simulink model "ErrorHandling_v2"  (R2020a)
settings: Solver=VariableStepAuto  StartTime=0.0  StopTime=10.0  RelTol=1e-3  EnableMultiTasking=on
settings Model: Creator=Flanker  LastModifiedBy=Flanker
settings DataIOCC: LimitDataPoints=on  ReturnWorkspaceOutputs=off
settings OptimizationCC: LifeSpan=inf
settings DebuggingCC: AllowSymbolicDim=off  SFUnexpectedBacktrackingDiag=warning  SFNoUnconditionalDefaultTransitionDiag=warning  SFExecutionAtInitializationDiag=none  ArithmeticOperatorsInVariantConditions=warning
settings ModelReferenceCC: PropagateSignalLabelsOutOfModel=off
settings SFSimCC: SimUseLocalCustomCode=off  CustomCodeUndefinedFunction=UseInterfaceOnly
settings RTWCC: RTWUseLocalCustomCode=off
settings CodeAppCC: StateflowObjectComments=on
settings GRTTargetCC: TargetLangStandard=C89/C90 (ANSI)
settings ConfigComp: CovMetricSettings=dw  CovHtmlReporting=on  CovSaveCumulativeToWorkspaceVar=on  CovSaveSingleToWorkspaceVar=on  CovExternalEMLEnable=off

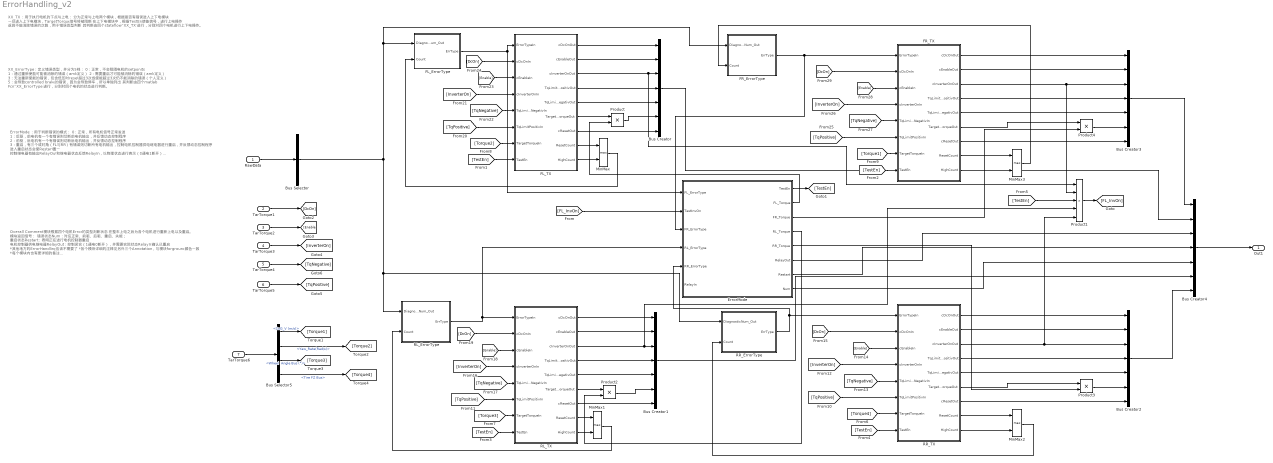
== system ErrorHandling_v2 ==
  note: XX_ErrorType ：定义错误类型，并分为5档：
      | 0：正常，不会阻隔电机的setponits
      | 1：通过重新使能可能被消除的错误（amk定义）
      | 2：需要重启才可能被消除的错误（amk定义）
      | 3：无法重新使能的错误，包含低压时reset超过3次或使能超过3次仍不能消除的错误（个人定义）
      | 5：会导致controlled brake的错误，因为会导致停车，所以单独列出
      |
      | 其判断由四个matlab Fcn“XX_ErrorType”进行，分别对四个电机的状态进行判断。
  note: XX_TX ：用于执行电机的下点与上电：
      | 分为正常与上电两个模块，根据是否有错误进入上下电模块
      | 一旦进入上下电模块，TargetTorque信号将被阻断
      | 在上下电模块中，根据TestEn使能信号，进行上电操作
      | 返回不能消除错误的次数，用于错误类型判断
      |
      | 其判断由四个stateflow“XX_TX”进行，分别对四个电机进行上下电操作。
  note: ErrorMode ：用于判断错误的模式：
      | 0：正常，所有电机信号正常发送
      | 1：后驱，前电机有一个有错误则切断前电机输出，并反馈动态控制程序
      | 2：前驱，后电机有一个有错误则切断后电机输出，并反馈动态控制程序
      | 3：重启，有三个或对角（FL与RR）有错误则切断所有电机输出，控制电机控制器供电继电器进行重启，并反馈动态控制程序
      | 进入重启状态会使Restart置一
      | 控制继电器有输出RelayOut和继电器状态反馈RelayIn，以物理状态进行表示（0通电1断开）
      | 电机控制器重新上电后，TestEn置一，控制TX模块进行电机上电
      | 4：失能，重启次数超过3次仍不能解除错误状态，则停止重启的状态，并反馈动态控制程序
      |
      | 会根据所在模式，切断TargetTorque信号
      |
      | 其判断由stateflow“ErrorMode”进行，分别对四个电机进行上下电操作。
  note: Overall Comment
      |
      | 模块根据四个电机Error的类型判断状态
      | 在整车上电之后为各个电机进行重新上电以及重启。
      |
      | 模块返回信号：
      |
      | 错误状态Num：对应正常、前驱、后驱、重启、失能；
      | 重启状态Restart：表明正在进行电机控制器重启
      | 电机控制器供电继电器RelayOut：控制闭合（1通电0断开），并需要实际状态RelayIn确认已重启
      |
      | *其他地方的ErrorHandling应该不需要了
      | *各个模块详细的注释见另外三个Annotation，与模块forground颜色一致
      | *每个模块内也有更详细的备注
      | *很多错误没有出现过，也没看懂到底怎么解决，所以归类方式以结果为主，并没有更深入的进行handling
      | *其实很多错误根本无法在行驶中被消除，但是垂死挣扎，此程序主要意义还是切换前驱后驱
      |
      | 2020/2/6 V2.0
  RawData : Inport
  TarTorque1 : Inport  Port=2
  TarTorque2 : Inport  Port=3
  TarTorque3 : Inport  Port=4
  TarTorque4 : Inport  Port=5
  TarTorque5 : Inport  Port=6
  TarTorque6 : Inport  Port=7
  Bus Creator{,1..4} (5 alike) : BusCreator  Inputs=7
  Bus Selector : BusSelector  OutputSignals=signal1,signal2  OutputAsBus=on
  Bus Selector5 : BusSelector  OutputSignals="processed data.CoG_V (m/s),processed data.Yaw_Rate(Rad/s),processed data.Wheel  Angle Bus (°),processed data.Tire FZ Bus"
  ErrorMode : Stateflow chart  TreatAsAtomicUnit=on
  FL_ErrorType : MATLAB Function  TreatAsAtomicUnit=on
  "FL_TX " : Stateflow chart  TreatAsAtomicUnit=on
  FR_ErrorType : MATLAB Function  TreatAsAtomicUnit=on
  FR_TX : Stateflow chart  TreatAsAtomicUnit=on
  MinMax{,1..3} (4 alike) : MinMax  Function=max  Inputs=2
  Product{,2..4} (4 alike) : Product
  Product1 : Product  Inputs=5
  RL_ErrorType : MATLAB Function  TreatAsAtomicUnit=on
  RL_TX : Stateflow chart  TreatAsAtomicUnit=on
  RR_ErrorType : MATLAB Function  TreatAsAtomicUnit=on
  RR_TX : Stateflow chart  TreatAsAtomicUnit=on
  Out1 : Outport
  wires:
  FL_ErrorType/1(ErrType) -> ErrorMode/1(FL_ErrorType), "FL_TX "/1(ErrorTypeIn)
  "FL_TX "/8(ResetCount) -> MinMax/1
  "FL_TX "/9(HighCount) -> MinMax/2
  MinMax/1 -> FL_ErrorType/2(Count)
  "FL_TX "/3(cInverterOnOut) -> Product1/1, Bus Creator/3
  "FL_TX "/1(cDcOnOut) -> Bus Creator/1
  "FL_TX "/2(cEnableOut) -> Bus Creator/2
  "FL_TX "/4(TqLimitPositivOut) -> Bus Creator/4
  "FL_TX "/5(TqLimitNegativOut) -> Bus Creator/5
  "FL_TX "/6(TargetTorqueOut) -> Product/1
  "FL_TX "/7(cResetOut) -> Bus Creator/7
  Product/1 -> Bus Creator/6
  [FL_InvOn] -> ErrorMode/2(TestInvOn)
  RawData/1 -> Bus Selector/1
  Product1/1 -> [FL_InvOn]
  RL_TX/3(cInverterOnOut) -> Product1/4, Bus Creator1/3
  RL_TX/1(cDcOnOut) -> Bus Creator1/1
  RL_TX/2(cEnableOut) -> Bus Creator1/2
  RL_TX/4(TqLimitPositivOut) -> Bus Creator1/4
  RL_TX/5(TqLimitNegativOut) -> Bus Creator1/5
  RL_TX/6(TargetTorqueOut) -> Product2/1
  RL_TX/7(cResetOut) -> Bus Creator1/7
  Product2/1 -> Bus Creator1/6
  RR_TX/3(cInverterOnOut) -> Bus Creator2/3, Product1/5
  RR_TX/1(cDcOnOut) -> Bus Creator2/1
  RR_TX/2(cEnableOut) -> Bus Creator2/2
  RR_TX/4(TqLimitPositivOut) -> Bus Creator2/4
  RR_TX/5(TqLimitNegativOut) -> Bus Creator2/5
  RR_TX/6(TargetTorqueOut) -> Product3/1
  RR_TX/7(cResetOut) -> Bus Creator2/7
  Product3/1 -> Bus Creator2/6
  FR_TX/3(cInverterOnOut) -> Bus Creator3/3, Product1/2
  FR_TX/1(cDcOnOut) -> Bus Creator3/1
  FR_TX/2(cEnableOut) -> Bus Creator3/2
  FR_TX/4(TqLimitPositivOut) -> Bus Creator3/4
  FR_TX/5(TqLimitNegativOut) -> Bus Creator3/5
  FR_TX/6(TargetTorqueOut) -> Product4/1
  FR_TX/7(cResetOut) -> Bus Creator3/7
  Product4/1 -> Bus Creator3/6
  FR_TX/8(ResetCount) -> MinMax3/1
  FR_TX/9(HighCount) -> MinMax3/2
  FR_ErrorType/1(ErrType) -> ErrorMode/3(FR_ErrorType), FR_TX/1(ErrorTypeIn)
  RL_TX/8(ResetCount) -> MinMax1/1
  RL_TX/9(HighCount) -> MinMax1/2
  RR_TX/8(ResetCount) -> MinMax2/1
  RR_TX/9(HighCount) -> MinMax2/2
  RR_ErrorType/1(ErrType) -> ErrorMode/5(RR_ErrorType), RR_TX/1(ErrorTypeIn)
  RL_ErrorType/1(ErrType) -> ErrorMode/4(RL_ErrorType), RL_TX/1(ErrorTypeIn)
  MinMax1/1 -> RL_ErrorType/2(Count)
  MinMax3/1 -> FR_ErrorType/2(Count)
  Bus Creator3/1 -> Bus Creator4/1
  Bus Creator/1 -> Bus Creator4/2
  Bus Creator1/1 -> Bus Creator4/6
  Bus Creator2/1 -> Bus Creator4/7
  Bus Creator4/1 -> Out1/1
  ErrorMode/1(TestEn) -> [TestEn]
  [TestEn] -> "FL_TX "/8(TestEn)
  [TestEn] -> FR_TX/8(TestEn)
  [TestEn] -> RL_TX/8(TestEn)
  [TestEn] -> Product1/3
  ErrorMode/2(FL_Torque) -> Product/2
  ErrorMode/3(FR_Torque) -> Product4/2
  ErrorMode/4(RL_Torque) -> Product2/2
  ErrorMode/5(RR_Torque) -> Product3/2
  ErrorMode/6(RelayOut) -> Bus Creator4/3
  ErrorMode/7(Restart) -> Bus Creator4/4
  Bus Selector/1 -> RL_ErrorType/1(DiagnosticNum_Out), RR_ErrorType/1(DiagnosticNum_Out), FR_ErrorType/1(DiagnosticNum_Out), FL_ErrorType/1(DiagnosticNum_Out)
  MinMax2/1 -> RR_ErrorType/2(Count)
  ErrorMode/8(Num) -> Bus Creator4/5
  TarTorque4/1 -> [TqNegative]
  TarTorque1/1 -> [DcOn]
  TarTorque2/1 -> [Enable]
  TarTorque3/1 -> [InverterOn]
  [TestEn] -> RR_TX/8(TestEn)
  TarTorque6/1 -> Bus Selector5/1
  Bus Selector5/2 -> [Torque2]  "<Yaw_Rate(Rad/s)>"
  Bus Selector5/1 -> [Torque1]  "<CoG_V (m/s)>"
  Bus Selector5/3 -> [Torque3]  "<Wheel  Angle Bus (°)>"
  Bus Selector5/4 -> [Torque4]  "<Tire FZ Bus>"
  [Torque4] -> RR_TX/7(TargetTorqueIn)
  [Torque3] -> RL_TX/7(TargetTorqueIn)
  [Torque2] -> "FL_TX "/7(TargetTorqueIn)
  [Torque1] -> FR_TX/7(TargetTorqueIn)
  TarTorque5/1 -> [TqPositive]
  [TqPositive] -> RR_TX/6(TqLimitPositivIn)
  [TqPositive] -> RL_TX/6(TqLimitPositivIn)
  [TqNegative] -> RR_TX/5(TqLimitNegativIn)
  [InverterOn] -> RR_TX/4(cInverterOnIn)
  [Enable] -> RR_TX/3(cEnableIn)
  [DcOn] -> RR_TX/2(cDcOnIn)
  [Enable] -> RL_TX/3(cEnableIn)
  [DcOn] -> RL_TX/2(cDcOnIn)
  [InverterOn] -> RL_TX/4(cInverterOnIn)
  [TqNegative] -> RL_TX/5(TqLimitNegativIn)
  [InverterOn] -> "FL_TX "/4(cInverterOnIn)
  [TqPositive] -> "FL_TX "/6(TqLimitPositivIn)
  [DcOn] -> "FL_TX "/2(cDcOnIn)
  [Enable] -> "FL_TX "/3(cEnableIn)
  [TqNegative] -> "FL_TX "/5(TqLimitNegativIn)
  [TqPositive] -> FR_TX/6(TqLimitPositivIn)
  [InverterOn] -> FR_TX/4(cInverterOnIn)
  [DcOn] -> FR_TX/2(cDcOnIn)
  [Enable] -> FR_TX/3(cEnableIn)
  [TqNegative] -> FR_TX/5(TqLimitNegativIn)

== stateflow chart ErrorHandling_v2/RL_TX ==
  state E1
    state S1
      en:
      TargetTorqueOut=0;
      TqLimitNegativOut=0;
      TqLimitPositivOut=0;
      n=0;
      du:
      n=n+1;
    state S8
      en:
      cInverterOn=1;
      n=0;
      du:
      n=n+1;
    state S2
      en:
      cInverterOnOut=0;
      n=0;
      du:
      n=n+1;
    state S7
      en:
      cEnableOut=1;
      n=0;
      du:
      n=n+1;
    state S3
      en:
      cEnableOut=0;
      n=0;
      du:
      n=n+1;
    state S6
      en:
      cDcOnOut=1;
      n=0;
      du:
      n=n+1;
    state S4
      en:
      cDcOnOut=0;
      n=0;
      du:
      n=n+1;
    state S5
      en:
      cReset=1;
      n=0;
      du:
      n=n+1;
      ex:
      cReset=0;
    (junction 68) -> S2 : HighCoun[ErrorTypeIn~=0]{HighCount = HighCount + 1;}
    S8 -> (junction 68) : [n>10]
    (default) -> S1
    S1 -> S2 : [n>5]
    S7 -> S8 : [n>5]
    S2 -> S3 : [n>5]
    S6 -> S7 : [n>5]
    (junction 85) -> S6 [order 2] : [TestEn==1]...
        | {HighCount=0;ResetCount=0;}
    S3 -> S4 : [n>5]
    (junction 43) -> S6 [order 1] : [ErrorTypeIn~=1]{ResetCount=0;}
    (junction 43) -> S5 [order 2] : ResetCoun[ErrorTypeIn==1&ResetCount<4]{ResetCount = ResetCount + 1;}
    (junction 43) -> (junction 85) [order 3] : [ResetCount==4]
    S5 -> (junction 43) : [n>10]
    S4 -> (junction 85) : [n>5]
  state E0
    en:
    ErrorState=ErrorTypeIn;
    ResetCount=0;
    HighCount=0;
    du:
    cDcOnOut=cDcOnIn;
    cEnableOut=cEnableIn;
    cInverterOnOut=cInverterOnIn;
    TqLimitPositivOut=TqLimitPositivIn;
    TqLimitNegativOut=TqLimitNegativIn;
    TargetTorqueOut=TargetTorqueIn;
    ex:
    ErrorState=ErrorTypeIn;
  note: TX ：用于执行电机的下电与上电：
      | 分为正常“E0”与上下电“E1”两个模块，根据是否有错误“ErrorTypeIn”进入上下电模块。
      | 一旦进入上下电模块，TqLimit以及TargetTorque信号将被阻断，并逐步下电。
      | 因为只有ErrorType=1时，下电再上电可能消除错误，其他错误类型（>1）将被限制在juncture处。
      | 当“ErrorMode”模块进行重启后，“TestEn”使上下电模块进行上电操作
      | “ResetCount”是低压错误重置失败次数，"HighCount"是使能后错误出现次数，两者将取最大值返回“XX_ErrorType”用于判断错误类型
      |
      | 注意：使用n计数可能导致命令送出时延过短（未成功送出），调试时需注意
  note: 
  (default) -> E0
  E0 -> E1 : [ErrorTypeIn~=0]
  E1 -> E0 : [ErrorTypeIn==0]
  (junction 85) -> S5 [order 1] : [ErrorTypeIn<2||HighCount<4]
  data: cDcOnOut output; ErrorTypeIn input; cDcOnIn input [0..1]; cEnableIn input [0..1]; cInverterOnIn input [0..1]; n local =0; cEnableOut output; cInverterOnOut output; TqLimitPositivOut output; TqLimitNegativOut output; TargetTorqueOut output; TqLimitNegativIn input; TqLimitPositivIn input; TargetTorqueIn input; cResetOut output; ErrorState local =0; ResetCount output =0; HighCount output =0; TestEn input

== matlab function ErrorHandling_v2/RL_ErrorType ==
  data: DiagnosticNum_Out input; ErrType output; Count input
function ErrType = ErrorType(DiagnosticNum_Out,Count)
    if DiagnosticNum_Out==0&&Count<4
        ErrType=0;%没有错误
    elseif (DiagnosticNum_Out==3587 || DiagnosticNum_Out==3585 ...
            ||MCFL_Diagnost==2310)&&Count<4
        ErrType=2;%错误需要软件重启
    elseif (DiagnosticNum_Out==1049 || DiagnosticNum_Out==1066 ...
            ||DiagnosticNum_Out==1101|| DiagnosticNum_Out==2360 ...
            ||DiagnosticNum_Out==2361|| DiagnosticNum_Out==2363 ...
            ||DiagnosticNum_Out==2364|| DiagnosticNum_Out==2365 ...
            ||DiagnosticNum_Out==2399)&&Count<4
        ErrType=4;%导致Controlled Brake的错误，停车进行硬件重启
    elseif DiagnosticNum_Out~=0&&Count>3
        ErrType=3;%无法重新使能的错误（由1、2产生）
    else
        ErrType = 1;%错误需要重新使能
    end
end
% 定义错误类型，并分为5档：
% 0：正常，不会阻隔电机的setponits
% 1：通过重新使能可能被消除的错误（amk定义），因为没被列举的错误极多，
% 很多没见过也不知如何处理，便用else归类
% 2：需要重启才可能被消除的错误（amk定义）
% 3：无法重新使能的错误，包含低压时reset超过3次或使能超过3次仍不能消除的错误（个人定义）
% 5：会导致controlled brake的错误，因为会导致停车，所以单独列出
% 
% 很多错误没有出现过，也没看懂到底怎么解决，所以归类方式以结果为主，并没有更深入的进行handling
% 其实很多错误根本无法在行驶中被消除，但是垂死挣扎，此程序主要意义还是切换前驱后驱

== stateflow chart ErrorHandling_v2/RR_TX ==
  state E1
    state S1
      en:
      TargetTorqueOut=0;
      TqLimitNegativOut=0;
      TqLimitPositivOut=0;
      n=0;
      du:
      n=n+1;
    state S8
      en:
      cInverterOn=1;
      n=0;
      du:
      n=n+1;
    state S2
      en:
      cInverterOnOut=0;
      n=0;
      du:
      n=n+1;
    state S7
      en:
      cEnableOut=1;
      n=0;
      du:
      n=n+1;
    state S3
      en:
      cEnableOut=0;
      n=0;
      du:
      n=n+1;
    state S6
      en:
      cDcOnOut=1;
      n=0;
      du:
      n=n+1;
    state S4
      en:
      cDcOnOut=0;
      n=0;
      du:
      n=n+1;
    state S5
      en:
      cReset=1;
      n=0;
      du:
      n=n+1;
      ex:
      cReset=0;
    (junction 68) -> S2 : HighCoun[ErrorTypeIn~=0]{HighCount = HighCount + 1;}
    S8 -> (junction 68) : [n>10]
    (default) -> S1
    S1 -> S2 : [n>5]
    S7 -> S8 : [n>5]
    S2 -> S3 : [n>5]
    S6 -> S7 : [n>5]
    (junction 85) -> S6 [order 2] : [TestEn==1]...
        | {HighCount=0;ResetCount=0;}
    S3 -> S4 : [n>5]
    (junction 43) -> S6 [order 1] : [ErrorTypeIn~=1]{ResetCount=0;}
    (junction 43) -> S5 [order 2] : ResetCoun[ErrorTypeIn==1&ResetCount<4]{ResetCount = ResetCount + 1;}
    (junction 43) -> (junction 85) [order 3] : [ResetCount==4]
    S5 -> (junction 43) : [n>10]
    S4 -> (junction 85) : [n>5]
  state E0
    en:
    ErrorState=ErrorTypeIn;
    ResetCount=0;
    HighCount=0;
    du:
    cDcOnOut=cDcOnIn;
    cEnableOut=cEnableIn;
    cInverterOnOut=cInverterOnIn;
    TqLimitPositivOut=TqLimitPositivIn;
    TqLimitNegativOut=TqLimitNegativIn;
    TargetTorqueOut=TargetTorqueIn;
    ex:
    ErrorState=ErrorTypeIn;
  note: TX ：用于执行电机的下电与上电：
      | 分为正常“E0”与上下电“E1”两个模块，根据是否有错误“ErrorTypeIn”进入上下电模块。
      | 一旦进入上下电模块，TqLimit以及TargetTorque信号将被阻断，并逐步下电。
      | 因为只有ErrorType=1时，下电再上电可能消除错误，其他错误类型（>1）将被限制在juncture处。
      | 当“ErrorMode”模块进行重启后，“TestEn”使上下电模块进行上电操作
      | “ResetCount”是低压错误重置失败次数，"HighCount"是使能后错误出现次数，两者将取最大值返回“XX_ErrorType”用于判断错误类型
      |
      | 注意：使用n计数可能导致命令送出时延过短（未成功送出），调试时需注意
  note: 
  (default) -> E0
  E0 -> E1 : [ErrorTypeIn~=0]
  E1 -> E0 : [ErrorTypeIn==0]
  (junction 85) -> S5 [order 1] : [ErrorTypeIn<2||HighCount<4]
  data: cDcOnOut output; ErrorTypeIn input; cDcOnIn input [0..1]; cEnableIn input [0..1]; cInverterOnIn input [0..1]; n local =0; cEnableOut output; cInverterOnOut output; TqLimitPositivOut output; TqLimitNegativOut output; TargetTorqueOut output; TqLimitNegativIn input; TqLimitPositivIn input; TargetTorqueIn input; cResetOut output; ErrorState local =0; ResetCount output =0; HighCount output =0; TestEn input

== matlab function ErrorHandling_v2/RR_ErrorType ==
  data: DiagnosticNum_Out input; ErrType output; Count input
function ErrType = ErrorType(DiagnosticNum_Out,Count)
    if DiagnosticNum_Out==0&&Count<4
        ErrType=0;%没有错误
    elseif (DiagnosticNum_Out==3587 || DiagnosticNum_Out==3585 ...
            ||MCFL_Diagnost==2310)&&Count<4
        ErrType=2;%错误需要软件重启
    elseif (DiagnosticNum_Out==1049 || DiagnosticNum_Out==1066 ...
            ||DiagnosticNum_Out==1101|| DiagnosticNum_Out==2360 ...
            ||DiagnosticNum_Out==2361|| DiagnosticNum_Out==2363 ...
            ||DiagnosticNum_Out==2364|| DiagnosticNum_Out==2365 ...
            ||DiagnosticNum_Out==2399)&&Count<4
        ErrType=4;%导致Controlled Brake的错误，停车进行硬件重启
    elseif DiagnosticNum_Out~=0&&Count>3
        ErrType=3;%无法重新使能的错误（由1、2产生）
    else
        ErrType = 1;%错误需要重新使能
    end
end
% 定义错误类型，并分为5档：
% 0：正常，不会阻隔电机的setponits
% 1：通过重新使能可能被消除的错误（amk定义），因为没被列举的错误极多，
% 很多没见过也不知如何处理，便用else归类
% 2：需要重启才可能被消除的错误（amk定义）
% 3：无法重新使能的错误，包含低压时reset超过3次或使能超过3次仍不能消除的错误（个人定义）
% 5：会导致controlled brake的错误，因为会导致停车，所以单独列出
% 
% 很多错误没有出现过，也没看懂到底怎么解决，所以归类方式以结果为主，并没有更深入的进行handling
% 其实很多错误根本无法在行驶中被消除，但是垂死挣扎，此程序主要意义还是切换前驱后驱

== stateflow chart ErrorHandling_v2/FR_TX ==
  state E1
    state S1
      en:
      TargetTorqueOut=0;
      TqLimitNegativOut=0;
      TqLimitPositivOut=0;
      n=0;
      du:
      n=n+1;
    state S8
      en:
      cInverterOn=1;
      n=0;
      du:
      n=n+1;
    state S2
      en:
      cInverterOnOut=0;
      n=0;
      du:
      n=n+1;
    state S7
      en:
      cEnableOut=1;
      n=0;
      du:
      n=n+1;
    state S3
      en:
      cEnableOut=0;
      n=0;
      du:
      n=n+1;
    state S6
      en:
      cDcOnOut=1;
      n=0;
      du:
      n=n+1;
    state S4
      en:
      cDcOnOut=0;
      n=0;
      du:
      n=n+1;
    state S5
      en:
      cReset=1;
      n=0;
      du:
      n=n+1;
      ex:
      cReset=0;
    (junction 68) -> S2 : HighCoun[ErrorTypeIn~=0]{HighCount = HighCount + 1;}
    S8 -> (junction 68) : [n>10]
    (default) -> S1
    S1 -> S2 : [n>5]
    S7 -> S8 : [n>5]
    S2 -> S3 : [n>5]
    S6 -> S7 : [n>5]
    (junction 85) -> S6 [order 2] : [TestEn==1]...
        | {HighCount=0;ResetCount=0;}
    S3 -> S4 : [n>5]
    (junction 43) -> S6 [order 1] : [ErrorTypeIn~=1]{ResetCount=0;}
    (junction 43) -> S5 [order 2] : ResetCoun[ErrorTypeIn==1&ResetCount<4]{ResetCount = ResetCount + 1;}
    (junction 43) -> (junction 85) [order 3] : [ResetCount==4]
    S5 -> (junction 43) : [n>10]
    S4 -> (junction 85) : [n>5]
  note: TX ：用于执行电机的下电与上电：
      | 分为正常“E0”与上下电“E1”两个模块，根据是否有错误“ErrorTypeIn”进入上下电模块。
      | 一旦进入上下电模块，TqLimit以及TargetTorque信号将被阻断，并逐步下电。
      | 因为只有ErrorType=1时，下电再上电可能消除错误，其他错误类型（>1）将被限制在juncture处。
      | 当“ErrorMode”模块进行重启后，“TestEn”使上下电模块进行上电操作
      | “ResetCount”是低压错误重置失败次数，"HighCount"是使能后错误出现次数，两者将取最大值返回“XX_ErrorType”用于判断错误类型
      |
      | 注意：使用n计数可能导致命令送出时延过短（未成功送出），调试时需注意
  state E0
    en:
    ErrorState=ErrorTypeIn;
    ResetCount=0;
    HighCount=0;
    du:
    cDcOnOut=cDcOnIn;
    cEnableOut=cEnableIn;
    cInverterOnOut=cInverterOnIn;
    TqLimitPositivOut=TqLimitPositivIn;
    TqLimitNegativOut=TqLimitNegativIn;
    TargetTorqueOut=TargetTorqueIn;
    ex:
    ErrorState=ErrorTypeIn;
  note: 
  (default) -> E0
  E0 -> E1 : [ErrorTypeIn~=0]
  E1 -> E0 : [ErrorTypeIn==0]
  (junction 85) -> S5 [order 1] : [ErrorTypeIn<2||HighCount<4]
  data: cDcOnOut output; ErrorTypeIn input; cDcOnIn input [0..1]; cEnableIn input [0..1]; cInverterOnIn input [0..1]; n local =0; cEnableOut output; cInverterOnOut output; TqLimitPositivOut output; TqLimitNegativOut output; TargetTorqueOut output; TqLimitNegativIn input; TqLimitPositivIn input; TargetTorqueIn input; cResetOut output; ErrorState local =0; ResetCount output =0; HighCount output =0; TestEn input

== matlab function ErrorHandling_v2/FR_ErrorType ==
  data: DiagnosticNum_Out input; ErrType output; Count input
function ErrType = ErrorType(DiagnosticNum_Out,Count)
     if DiagnosticNum_Out==0&&Count<4
         ErrType=0;% no error
     elseif (DiagnosticNum_Out==3587 || DiagnosticNum_Out==3585 ...
             ||MCFL_Diagnost==2310)&&Count<4
         ErrType=2;% error requires software restart
     elseif (DiagnosticNum_Out==1049 || DiagnosticNum_Out==1066 ...
             ||DiagnosticNum_Out==1101|| DiagnosticNum_Out==2360 ...
             ||DiagnosticNum_Out==2361|| DiagnosticNum_Out==2363 ...
             ||DiagnosticNum_Out==2364|| DiagnosticNum_Out==2365 ...
             ||DiagnosticNum_Out==2399)&&Count<4
         ErrType=4;% causes Controlled Brake error, stop and restart the hardware
     elseif DiagnosticNum_Out~=0&&Count>3
         ErrType=3;% error that cannot be re-enabled (generated by 1, 2)
     else
         ErrType = 1;% error needs to be re-enabled
     end
end
% Define the error type and divide it into 5 levels:
% 0: normal, will not block the setponits of the motor
% 1: Errors that may be eliminated by re-enabling (amk definition), 
% because there are so many errors that are not listed.
% Many people who haven’t seen it and don’t know how to deal with it, use else to classify
% 2: Errors that may be eliminated only after restarting (amk definition)
% 3: Errors that cannot be re-enabled, including errors that cannot be 
% eliminated after resetting more than 3 times or enabling more than 3 times under low voltage (personal definition)
% 5: Will cause the error of controlled brake, because it will cause parking, so it is listed separately
%
% Many errors have not appeared before, and I have not understood how to solve them, 
% so the classification method is based on the results, and there is no more in-depth handling
% In fact, many errors cannot be eliminated while driving, but they are struggling. 
% The main meaning of this program is to switch front and rear drives.

== matlab function ErrorHandling_v2/FL_ErrorType ==
  data: DiagnosticNum_Out input; ErrType output; Count input
function ErrType = ErrorType(DiagnosticNum_Out,Count)
    if DiagnosticNum_Out==0&&Count<4
        ErrType=0;%没有错误
    elseif (DiagnosticNum_Out==3587 || DiagnosticNum_Out==3585 ...
            ||MCFL_Diagnost==2310)&&Count<4
        ErrType=2;%错误需要软件重启
    elseif (DiagnosticNum_Out==1049 || DiagnosticNum_Out==1066 ...
            ||DiagnosticNum_Out==1101|| DiagnosticNum_Out==2360 ...
            ||DiagnosticNum_Out==2361|| DiagnosticNum_Out==2363 ...
            ||DiagnosticNum_Out==2364|| DiagnosticNum_Out==2365 ...
            ||DiagnosticNum_Out==2399)&&Count<4
        ErrType=4;%导致Controlled Brake的错误，停车进行硬件重启
    elseif DiagnosticNum_Out~=0&&Count>3
        ErrType=3;%无法重新使能的错误（由1、2产生）
    else
        ErrType = 1;%错误需要重新使能
    end
end
% 定义错误类型，并分为5档：
% 0：正常，不会阻隔电机的setponits
% 1：通过重新使能可能被消除的错误（amk定义），因为没被列举的错误极多，
% 很多没见过也不知如何处理，便用else归类
% 2：需要重启才可能被消除的错误（amk定义）
% 3：无法重新使能的错误，包含低压时reset超过3次或使能超过3次仍不能消除的错误（个人定义）
% 5：会导致controlled brake的错误，因为会导致停车，所以单独列出
% 
% 很多错误没有出现过，也没看懂到底怎么解决，所以归类方式以结果为主，并没有更深入的进行handling
% 其实很多错误根本无法在行驶中被消除，但是垂死挣扎，此程序主要意义还是切换前驱后驱

== stateflow chart ErrorHandling_v2/ErrorMode ==
  state Restart
    state S2
      en:
      TestEn=1;
      ex:
      TestEn=0;
      Restart=0;
    state R1
      en:
      RelayOut=0;
      Restart=1；
      ex:
      RelayOut=1;
    (default) -> R1
    (junction 32) -> (junction 36) : after(10,sec)
    (junction 36) -> S2
    R1 -> (junction 32) : [RelayIn==0]
    S2 -> R1 [order 4] : [N==3&&(RestartCount<4)...
        | &&InvOnOut==1]...
        | {RestartCount = RestartCount + 1;}
  state WD4
    en:
    Restart=0;
    du:
    FL_Torque=1;
    FR_Torque=1;
    RL_Torque=1;
    RR_Torque=1;
  note: ErrorMode ：The mode used to judge the error:
      | The judgment of the mode is done by MatlabFcn "Num":
      | Num=0: "WD4" is normal, all motor signals are sent normally
      | Num=1: "RED" rear drive, if there is an error in the front motor, the output of the front motor will be cut off
      | Num=2: "FWD" front drive, if there is an error in the rear motor, cut off the output of the rear motor
      | Num=3: "Restart" restarts, if there are three or diagonal (FL and RR) errors, cut off all motor outputs and control the motor controller power supply relay to restart
      | Entering the restart state will set "Restart" to one (Reserved has no actual use defined for the time being)
      | The control relay has output "RelayOut" and relay status feedback "RelayIn", which are represented by physical status (1 power on and 0 off)
      | After restarting, it takes a certain time (about 7s) for the motor controller to initialize, so the next steps will be delayed for 10s.
      | The motor controller restarts, "TestEn" is set to 1, and the TX module is controlled to power on the motor: the TX module is restricted to the unpowered state (all setpoints=0) due to an error. "TestEn" is used to test and power on. After power-on ("InvOnOut", derived from the last command when the four motors are powered on) Num changes, you can switch to other states. This is used to prevent error-free power on at low voltage
      | Num=4: Disabled, staying in S2 of Restart: Restarting times "RestartCount" more than 3 times can not clear the error state, then stop restarting state
      |
      | According to the mode, the "XX_Torque" output cuts off the TargetTorque signal;
      | Num is output at the same time to assist the dynamic control algorithm to switch torque distribution
  state FWD
    du:
    FL_Torque=1;
    FR_Torque=1;
    RL_Torque=0;
    RR_Torque=0;
  state RWD
    du:
    FL_Torque=0;
    FR_Torque=0;
    RL_Torque=1;
    RR_Torque=1;
  S2 -> WD4 [order 1] : [Num==0&&InvOnOut==1]{RestartCount=0;}
  (default) -> WD4
  WD4 -> Restart [order 3] : [Num==3]
  WD4 -> FWD [order 2] : [Num==2]
  WD4 -> RWD [order 1] : [Num==1]
  S2 -> FWD [order 3] : [Num==2&&InvOnOut==1]{RestartCount=0;}
  S2 -> RWD [order 2] : [Num==1&&InvOnOut==1]{RestartCount=0;}
  FWD -> Restart [order 2] : [Num==3]
  RWD -> Restart [order 2] : [Num==3]
  FWD -> WD4 [order 1] : [Num==0]
  RWD -> WD4 [order 1] : [Num==0]
  data: FL_ErrorType input; TestInvOn input; FR_ErrorType input; RL_ErrorType input; RR_ErrorType input; TestEn output boolean =0; FL_Torque output boolean =1; FR_Torque output boolean =1; RL_Torque output boolean =1; RR_Torque output boolean =1; n local uint8; RelayIn input; RelayOut output boolean; RestartCount local; Restart output boolean; Num output
  function Num:
    | function Num=Mode(FL_ErrorType,FR_ErrorType,RL_ErrorType,RR_ErrorType,RestartCount)
    | if FL_ErrorType==0&&FR_ErrorType==0&&...
    |         RL_ErrorType==0&&RR_ErrorType==0
    |     Num=0;%正常
    | elseif (FL_ErrorType==1||FR_ErrorType==1)&&...
    |         RL_ErrorType==0&&RR_ErrorType==0
    |     Num=1;%后驱
    | elseif (RL_ErrorType==1||RR_ErrorType==1)&&...
    |         FL_ErrorType==0&&FR_ErrorType==0
    |     Num=2;%前驱
    | elseif ((FL_ErrorType==1&&RR_ErrorType==1)||...
    |         (FR_ErrorType==1&&RL_ErrorType==1))&&...
    |         RestartCount<4
    |     Num=3;%需要进行重启
    | else
    |     Num=4;%失能（重启失败（3次以上））
    | end
    | end

== stateflow chart ErrorHandling_v2/FL_TX  ==
  state E1
    state S1
      en:
      TargetTorqueOut=0;
      TqLimitNegativOut=0;
      TqLimitPositivOut=0;
      n=0;
      du:
      n=n+1;
    state S8
      en:
      cInverterOn=1;
      n=0;
      du:
      n=n+1;
    state S2
      en:
      cInverterOnOut=0;
      n=0;
      du:
      n=n+1;
    state S7
      en:
      cEnableOut=1;
      n=0;
      du:
      n=n+1;
    state S3
      en:
      cEnableOut=0;
      n=0;
      du:
      n=n+1;
    state S6
      en:
      cDcOnOut=1;
      n=0;
      du:
      n=n+1;
    state S4
      en:
      cDcOnOut=0;
      n=0;
      du:
      n=n+1;
    state S5
      en:
      cReset=1;
      n=0;
      du:
      n=n+1;
      ex:
      cReset=0;
    (junction 68) -> S2 : HighCoun[ErrorTypeIn~=0]{HighCount = HighCount + 1;}
    S8 -> (junction 68) : [n>10]
    (default) -> S1
    S1 -> S2 : [n>5]
    S7 -> S8 : [n>5]
    S2 -> S3 : [n>5]
    S6 -> S7 : [n>5]
    (junction 85) -> S6 [order 2] : [TestEn==1]...
        | {HighCount=0;ResetCount=0;}
    S3 -> S4 : [n>5]
    (junction 43) -> S6 [order 1] : [ErrorTypeIn~=1]{ResetCount=0;}
    (junction 43) -> S5 [order 2] : ResetCoun[ErrorTypeIn==1&ResetCount<4]{ResetCount = ResetCount + 1;}
    (junction 43) -> (junction 85) [order 3] : [ResetCount==4]
    S5 -> (junction 43) : [n>10]
    S4 -> (junction 85) : [n>5]
    (junction 85) -> S5 [order 1] : [ErrorTypeIn<2||HighCount<4]
  note: TX ：Used to power off and power on the motor:
      | It is divided into two modules: normal "E0" and power-on and power-on "E1", and enters the power-on and power-off modules according to whether there is an error "ErrorTypeIn".
      | Once in the power-on and power-off module, the TqLimit and TargetTorque signals will be blocked and the power will be gradually powered off.
      | Because only when ErrorType=1, the error may be eliminated after power-off and power-on, and other error types (>1) will be limited to juncture.
      | When the "ErrorMode" module restarts, "TestEn" makes the power-on and power-off module perform power-on operations
      | "ResetCount" is the number of low-voltage error reset failures, "HighCount" is the number of error occurrences after enabling, the two will take the maximum value and return "XX_ErrorType" to determine the error type
      |
      | Note: Using n to count may result in too short command sending delay (unsuccessful sending), please pay attention when debugging
  state E0
    en:
    ErrorState=ErrorTypeIn;
    ResetCount=0;
    HighCount=0;
    du:
    cDcOnOut=cDcOnIn;
    cEnableOut=cEnableIn;
    cInverterOnOut=cInverterOnIn;
    TqLimitPositivOut=TqLimitPositivIn;
    TqLimitNegativOut=TqLimitNegativIn;
    TargetTorqueOut=TargetTorqueIn;
    ex:
    ErrorState=ErrorTypeIn;
  note: 
  (default) -> E0
  E0 -> E1 : [ErrorTypeIn~=0]
  E1 -> E0 : [ErrorTypeIn==0]
  data: cDcOnOut output; ErrorTypeIn input; cDcOnIn input [0..1]; cEnableIn input [0..1]; cInverterOnIn input [0..1]; n local =0; cEnableOut output; cInverterOnOut output; TqLimitPositivOut output; TqLimitNegativOut output; TargetTorqueOut output; TqLimitNegativIn input; TqLimitPositivIn input; TargetTorqueIn input; cResetOut output; ErrorState local =0; ResetCount output =0; HighCount output =0; TestEn input
